simulink model "NetworkModelSimpleIntersectionCRCA"  (R2018b)
settings: Solver=VariableStepAuto  StartTime=tStart  StopTime=tFinal  FixedStep=0.001  RelTol=1e-3
values from neighbouring files (symbols this model uses):
  Ax = [0 1  0   0 ... (first row only)    [DroneSubsystemModelling.m]
  Ay = [0 1  0   0 ... (first row only)    [DroneSubsystemModelling.m]
  Bx = [0;0;0;b1]    [DroneSubsystemModelling.m]
  By = [0;0;0;b2]    [DroneSubsystemModelling.m]
  ConflictDrone2andDrone4 = ControlDetectionFunction(tout,PositionXDrone2, PositionYDrone2, PositionXDrone4, PositionYDrone4, ConflictDrone2andDrone4)    [ConflictDetection.m]    (also in ConflictDetectionTEST.m = ControlDetectionFunction(tout,PositionXDrone2TEST, PositionY)
  Cpx = [1 0 0 0]    [DroneSubsystemModelling.m]
  Cpy = [1 0 0 0]    [DroneSubsystemModelling.m]
  Cvx = [0 1 0 0]    [DroneSubsystemModelling.m]
  Cvy = [0 1 0 0]    [DroneSubsystemModelling.m]
  theta2 = -3*180/4    (= -135)    [MotionModelling.m]
  theta4 = -180/4    (= -45)    [MotionModelling.m]
  VelocityStarX2 = vx20    [MotionModelling.m]
  VelocityStarX4 = vx40    [MotionModelling.m]
  VelocityStarY2 = vy20    [MotionModelling.m]
  VelocityStarY4 = vy40    [MotionModelling.m]
  X20 = [x20 vx20 0 0]'    [MotionModelling.m]
  X40 = [x40 vx40 0 0]'    [MotionModelling.m]
  Y20 = [y20 vy20 0 0]'    [MotionModelling.m]
  Y40 = [y40 vy40 0 0]'    [MotionModelling.m]
libraries: simulink x4
settings Model: Creator=CowUser  LastModifiedBy=CowUser

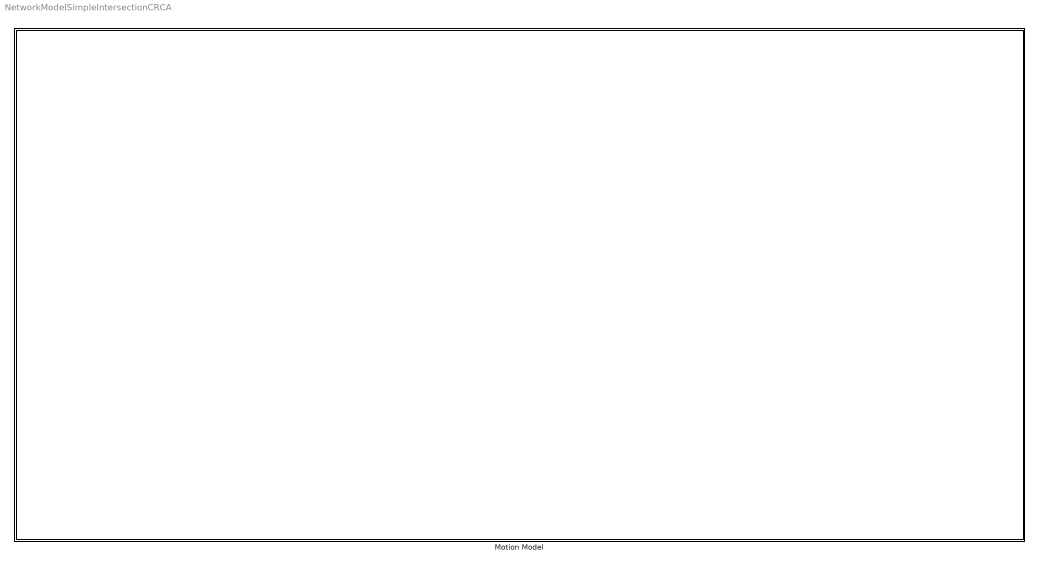
== system NetworkModelSimpleIntersectionCRCA ==
  Motion Model : Subsystem

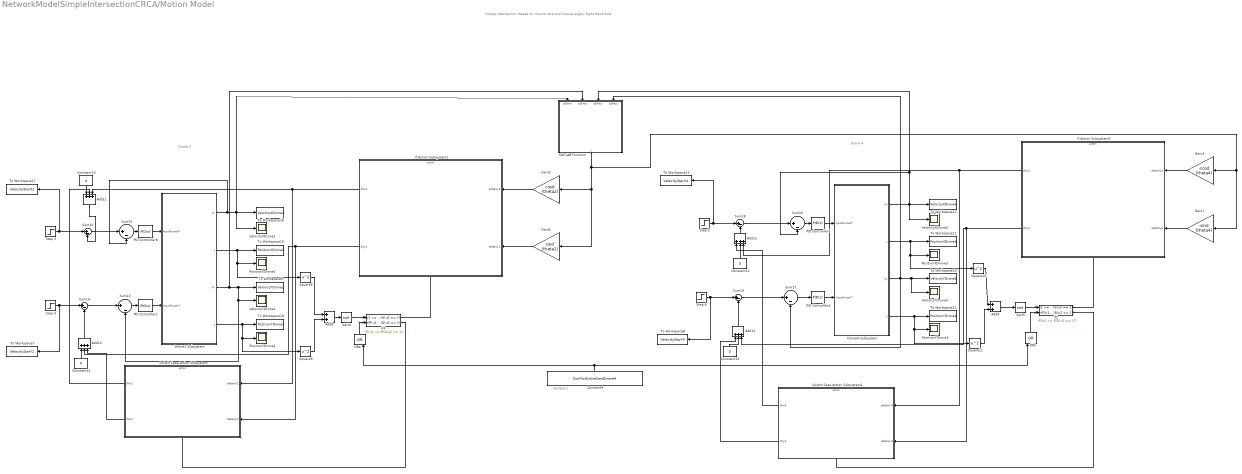
== system NetworkModelSimpleIntersectionCRCA/Motion Model ==
  note: Drone 4
  note: Drone 2
  note: Sample 1
  note: Simple Intersection
      | (based on closure rate and closure angle)
      |
      | Right Hand Rule
  Add{10..13} (4 alike) : Sum  Inputs=+++
  Add8 : Sum
  Add9 : Sum
  Constant{10..13} (4 alike) : Constant  Value=0
  Constant9 : Constant  Value=ConflictDrone2andDrone4
  Drone2 Subsystem : Subsystem
  Drone4 Subsystem : Subsystem
  Gain1 : Gain  Gain=-sind (theta4)
  Gain2 : Gain  Gain=cosd (theta2)
  Gain3 : Gain  Gain=-cosd (theta4)
  Gain4 : Gain  Gain=sind (theta2)
  If Action Subsystem2 : Subsystem  TreatAsAtomicUnit=on
  If Action Subsystem3 : Subsystem  TreatAsAtomicUnit=on
  If2 : If  NumInputs=2  IfExpression=(u1 <= R)&(u2 == 1)  ElseIfExpressions=(u1 > R)&(u2 == 1)  ShowElse=off
  If4 : If  NumInputs=2  IfExpression=(u1 <= R)&(u2 == 1)  ElseIfExpressions=(u1 > R)&(u2 == 1)  ShowElse=off
  MATLAB Function : MATLAB Function  TreatAsAtomicUnit=on
  OR3 : Logic  Operator=OR  Inputs=3  IconShape=distinctive  AllPortsSameDT=off  OutDataTypeStr='double'
  OR4 : Logic  Operator=OR  Inputs=3  IconShape=distinctive  AllPortsSameDT=off  OutDataTypeStr='double'
  PID Controller{2,4..5,8} (4 alike) : simulink/Continuous/PID Controller  Controller=PID  Form=Parallel  TimeDomain=Continuous-time  SampleTime=-1  IntegratorMethod=Forward Euler  FilterMethod=Forward Euler  ControllerParametersSource=internal  P=1.97139727738968e-05  I=1.5233344900537e-08  D=0.00566857635684116  UseFilter=on  N=15.1370363747334  TunerSelectOption=Transfer Function Based (PID Tuner App)  InitialConditionSource=internal  InitialConditionForIntegrator=0  InitialConditionForFilter=0  DifferentiatorICPrevScaledInput=0  ExternalReset=none  TrackingMode=off  Kt=1  LimitOutput=off  UpperSaturationLimit=inf  LowerSaturationLimit=-inf  LinearizeAsGain=on  AntiWindupMode=none  Kb=1  POutMin=[]  POutMax=[]  IOutMin=[]  IOutMax=[]  DOutMin=[]  DOutMax=[]  NOutMin=[]  NOutMax=[]  SumOutMin=[]  SumOutMax=[]  SaturationOutMin=[]  SaturationOutMax=[]  PParamMin=[]  PParamMax=[]  IParamMin=[]  IParamMax=[]  DParamMin=[]  DParamMax=[]  NParamMin=[]  NParamMax=[]  KbParamMin=[]  KbParamMax=[]  KtParamMin=[]  KtParamMax=[]  KbOutMin=[]  KbOutMax=[]  KtOutMin=[]  KtOutMax=[]  IntegratorOutMin=[]  IntegratorOutMax=[]  FilterOutMin=[]  FilterOutMax=[]  SumI1OutMin=[]  SumI1OutMax=[]  SumI2OutMin=[]  SumI2OutMax=[]  SumI3OutMin=[]  SumI3OutMax=[]  SumI4OutMin=[]  SumI4OutMax=[]  SumDOutMin=[]  SumDOutMax=[]  DifferentiatorOutMin=[]  DifferentiatorOutMax=[]  FilterDiffOutCoefMin=[]  FilterDiffOutCoefMax=[]  ReciprocalOutMin=[]  ReciprocalOutMax=[]  SumDenOutMin=[]  SumDenOutMax=[]  SumNumOutMin=[]  SumNumOutMax=[]  DivideOutMin=[]  DivideOutMax=[]  IntegratorContinuousStateAttributes=''  IntegratorStateMustResolveToSignalObject=off  IntegratorRTWStateStorageClass=Auto  FilterContinuousStateAttributes=''  FilterStateMustResolveToSignalObject=off  FilterRTWStateStorageClass=Auto  ParallelPVariant=InternalParameters  IdealPVariant=Disabled  IVariant=InternalParameters  DVariant=InternalParameters  IntegratorVariant=Continuous  SatVariant=Disabled  AWVariant=Passthrough  PCopyVariant=Disabled  TRVariant=Disabled  FdbkBlocksVariant=Forward  IdealPFdbkVariant=Disabled  SatFdbkVariant=Disabled  DerivativeFilterVariant=ContFilter  NVariant=InternalParameters  NCopyVariant=Disabled  FilterICVariant=InternalICsFilter  IntegratorICVariant=InternalICs  ExternalResetVariant=Disabled  TRSumVariant=Passthrough  SumFdbkVariant=Disabled  SumVariant=Sum_PID
  PositionXDrone1 : Scope
  PositionXDrone3 : Scope
  PositionYDrone1 : Scope
  PositionYDrone3 : Scope
  Sqrt4 : Sqrt  SaturateOnIntegerOverflow=on
  Sqrt5 : Sqrt  SaturateOnIntegerOverflow=on
  Square{8..11} (4 alike) : Math  Operator=square  SaturateOnIntegerOverflow=on
  Step 3 : Step  Time=0  After=VelocityStarX2  SampleTime=0
  Step 4 : Step  Time=0  After=VelocityStarY2  SampleTime=0
  Step 5 : Step  Time=0  After=VelocityStarX4  SampleTime=0
  Step 6 : Step  Time=0  After=VelocityStarY4  SampleTime=0
  Sum{13..20} (8 alike) : Sum  Inputs=|+-
  Switch Case Action Subsystem : Subsystem  TreatAsAtomicUnit=on
  Switch Case Action Subsystem1 : Subsystem  TreatAsAtomicUnit=on
  To Workspace10 : ToWorkspace  VariableName=VelocityYDrone4  SampleTime=-1
  To Workspace11 : ToWorkspace  VariableName=PositionXDrone4  SampleTime=-1
  To Workspace12 : ToWorkspace  VariableName=VelocityXDrone4  SampleTime=-1
  To Workspace13 : ToWorkspace  VariableName=VelocityStarX4  SampleTime=-1
  To Workspace14 : ToWorkspace  VariableName=PositionYDrone4  SampleTime=-1
  To Workspace15 : ToWorkspace  VariableName=PositionXDrone2  SampleTime=-1
  To Workspace16 : ToWorkspace  VariableName=VelocityXDrone2  SampleTime=-1
  To Workspace17 : ToWorkspace  VariableName=VelocityStarX2  SampleTime=-1
  To Workspace18 : ToWorkspace  VariableName=PositionYDrone2  SampleTime=-1
  To Workspace7 : ToWorkspace  VariableName=VelocityStarY2  SampleTime=-1
  To Workspace8 : ToWorkspace  VariableName=VelocityStarY4  SampleTime=-1
  To Workspace9 : ToWorkspace  VariableName=VelocityYDrone2  SampleTime=-1
  VelocityXDrone1 : Scope
  VelocityXDrone3 : Scope
  VelocityYDrone1 : Scope
  VelocityYDrone3 : Scope
  wires:
  Square10/1 -> Add9/1
  PID Controller2/1 -> Drone2 Subsystem/2("InputForceY* ")
  Sqrt4/1 -> If4/1
  Step 6/1 -> To Workspace8/1, Sum19/1
  Sum15/1 -> PID Controller8/1
  Gain2/1 -> If Action Subsystem2/1(deltaVx2)
  Step 4/1 -> Sum14/1, To Workspace7/1
  Constant9/1 -> OR4/3, OR3/1
  If Action Subsystem2/2(dVy2) -> Add10/2, Switch Case Action Subsystem/2(deltaVy2)
  Sqrt5/1 -> If2/1
  Sum16/1 -> PID Controller5/1
  If Action Subsystem3/1(dVx4) -> Switch Case Action Subsystem1/1(deltaVx4), Add12/3
  Constant10/1 -> Add11/2
  Constant13/1 -> Add13/2
  If Action Subsystem3/2(dVy4) -> Switch Case Action Subsystem1/2(deltaVy4), Add13/3
  Sum20/1 -> Sum15/1
  Add10/1 -> Sum14/2
  Drone2 Subsystem/3(Vy) -> To Workspace9/1, Sum13/2, VelocityYDrone1/1, MATLAB Function/2(qDotxj)
  PID Controller5/1 -> Drone4 Subsystem/1(InputForceX*)
  Switch Case Action Subsystem/2(dVy2) -> Add10/3
  Switch Case Action Subsystem/1(dVx2) -> Add11/1
  If4/1 -> If Action Subsystem2/Action
  Step 3/1 -> Sum20/1, To Workspace17/1
  Add11/1 -> Sum20/2
  Sum19/1 -> Sum17/1
  Sum14/1 -> Sum13/1
  Gain3/1 -> If Action Subsystem3/1(deltaVx4)
  Constant11/1 -> Add10/1
  Gain4/1 -> If Action Subsystem2/2(deltaVy2)
  OR4/1 -> If4/2
  Step 5/1 -> Sum18/1, To Workspace13/1
  Constant12/1 -> Add12/2
  Drone4 Subsystem/4(y) -> Square11/1, PositionYDrone3/1, To Workspace14/1
  If2/2 -> Switch Case Action Subsystem1/Action
  Square9/1 -> Add8/2
  Square8/1 -> Add8/1
  Add9/1 -> Sqrt5/1
  Switch Case Action Subsystem1/2(dVy4) -> Add13/1
  Sum17/1 -> PID Controller4/1
  Square11/1 -> Add9/2
  If2/1 -> If Action Subsystem3/Action
  Add13/1 -> Sum19/2
  Sum13/1 -> PID Controller2/1
  PID Controller8/1 -> Drone2 Subsystem/1(InputForceX*)
  OR3/1 -> If2/2
  If4/2 -> Switch Case Action Subsystem/Action
  Add12/1 -> Sum18/2
  Drone4 Subsystem/2(x) -> Square10/1, PositionXDrone3/1, To Workspace11/1
  Gain1/1 -> If Action Subsystem3/2(deltaVy4)
  Add8/1 -> Sqrt4/1
  Drone2 Subsystem/2(x) -> Square8/1, PositionXDrone1/1, To Workspace15/1
  MATLAB Function/1(y) -> Gain4/1, Gain2/1, Gain3/1, Gain1/1
  Drone4 Subsystem/1(Vx) -> MATLAB Function/3(qDotyi), Sum16/2, To Workspace12/1, VelocityXDrone3/1
  If Action Subsystem2/1(dVx2) -> Switch Case Action Subsystem/1(deltaVx2), Add11/3
  Drone2 Subsystem/4(y) -> To Workspace18/1, Square9/1, PositionYDrone1/1
  PID Controller4/1 -> Drone4 Subsystem/2("InputForceY* ")
  Drone4 Subsystem/3(Vy) -> MATLAB Function/4(qDotyj), Sum17/2, VelocityYDrone3/1, To Workspace10/1
  Sum18/1 -> Sum16/1
  Switch Case Action Subsystem1/1(dVx4) -> Add12/1
  Drone2 Subsystem/1(Vx) -> Sum15/2, MATLAB Function/1(qDotxi), VelocityXDrone1/1, To Workspace16/1

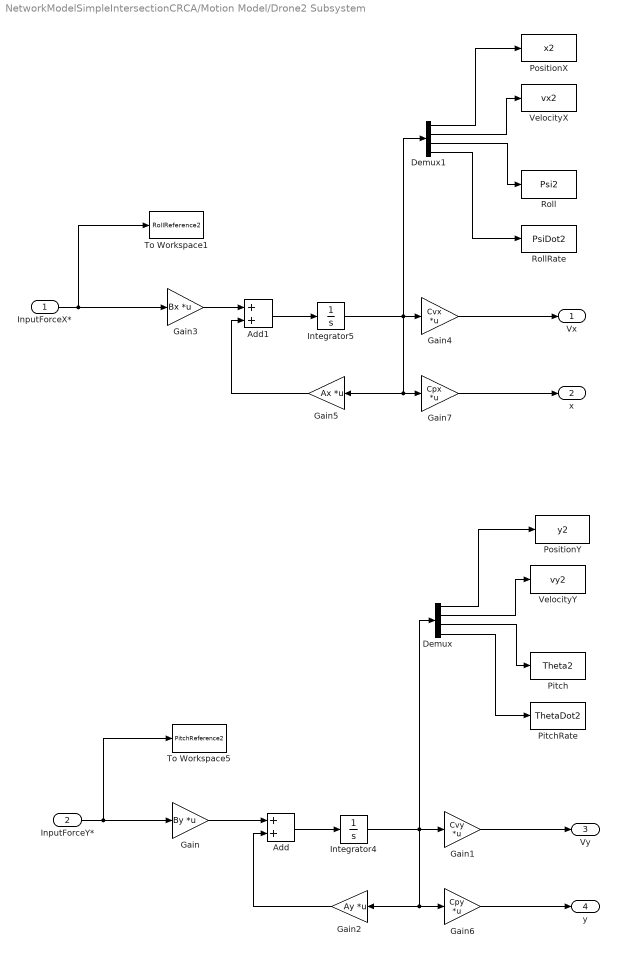
== system NetworkModelSimpleIntersectionCRCA/Motion Model/Drone2 Subsystem ==
  InputForceX* : Inport
  "InputForceY* " : Inport  Port=2
  Add : Sum
  Add1 : Sum
  Demux : Demux
  Demux1 : Demux
  Gain : Gain  Gain=By  Multiplication=Matrix(K*u)
  Gain1 : Gain  Gain=Cvy  Multiplication=Matrix(K*u)
  Gain2 : Gain  Gain=Ay  Multiplication=Matrix(K*u)
  Gain3 : Gain  Gain=Bx  Multiplication=Matrix(K*u)
  Gain4 : Gain  Gain=Cvx  Multiplication=Matrix(K*u)
  Gain5 : Gain  Gain=Ax  Multiplication=Matrix(K*u)
  Gain6 : Gain  Gain=Cpy  Multiplication=Matrix(K*u)
  Gain7 : Gain  Gain=Cpx  Multiplication=Matrix(K*u)
  Integrator4 : Integrator  InitialCondition=Y20
  Integrator5 : Integrator  InitialCondition=X20
  Pitch : ToWorkspace  VariableName=Theta2  SampleTime=-1
  PitchRate : ToWorkspace  VariableName=ThetaDot2  SampleTime=-1
  PositionX : ToWorkspace  VariableName=x2  SampleTime=-1
  PositionY : ToWorkspace  VariableName=y2  SampleTime=-1
  Roll : ToWorkspace  VariableName=Psi2  SampleTime=-1
  RollRate : ToWorkspace  VariableName=PsiDot2  SampleTime=-1
  To Workspace1 : ToWorkspace  VariableName=RollReference2  SampleTime=-1
  To Workspace5 : ToWorkspace  VariableName=PitchReference2  SampleTime=-1
  VelocityX : ToWorkspace  VariableName=vx2  SampleTime=-1
  VelocityY : ToWorkspace  VariableName=vy2  SampleTime=-1
  Vx : Outport
  x : Outport  Port=2
  Vy : Outport  Port=3
  y : Outport  Port=4
  wires:
  Demux/1 -> PositionY/1
  Demux1/2 -> VelocityX/1
  Demux1/4 -> RollRate/1
  Demux1/3 -> Roll/1
  Gain4/1 -> Vx/1
  "InputForceY* "/1 -> Gain/1, To Workspace5/1
  Gain/1 -> Add/1
  Demux/4 -> PitchRate/1
  Demux/3 -> Pitch/1
  Add/1 -> Integrator4/1
  Demux1/1 -> PositionX/1
  Gain1/1 -> Vy/1
  InputForceX*/1 -> Gain3/1, To Workspace1/1
  Gain7/1 -> x/1
  Integrator4/1 -> Gain6/1, Gain2/1, Demux/1, Gain1/1
  Demux/2 -> VelocityY/1
  Gain6/1 -> y/1
  Gain3/1 -> Add1/1
  Add1/1 -> Integrator5/1
  Gain2/1 -> Add/2
  Integrator5/1 -> Gain4/1, Gain5/1, Gain7/1, Demux1/1
  Gain5/1 -> Add1/2

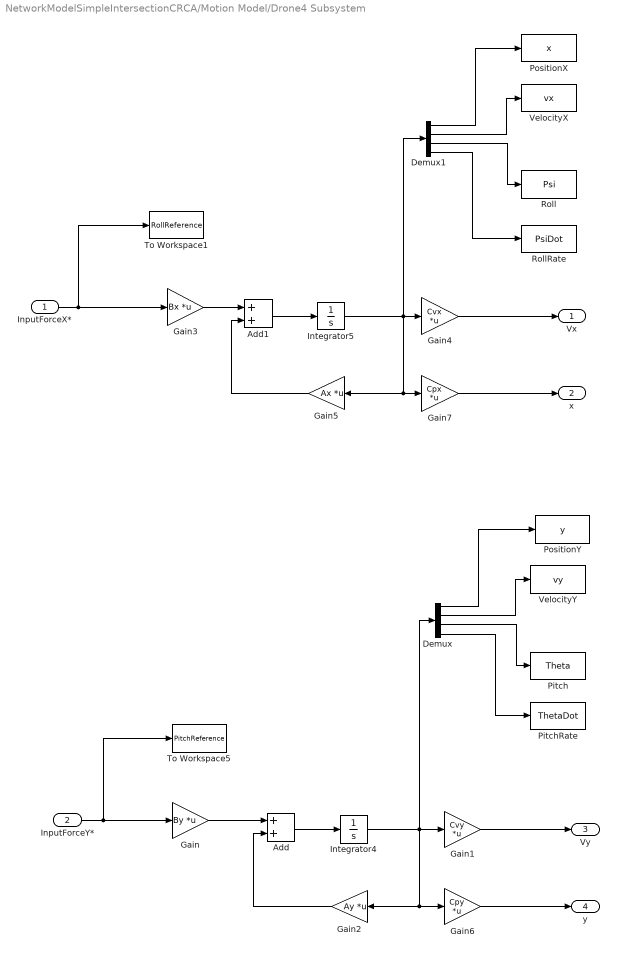
== system NetworkModelSimpleIntersectionCRCA/Motion Model/Drone4 Subsystem ==
  InputForceX* : Inport
  "InputForceY* " : Inport  Port=2
  Add : Sum
  Add1 : Sum
  Demux : Demux
  Demux1 : Demux
  Gain : Gain  Gain=By  Multiplication=Matrix(K*u)
  Gain1 : Gain  Gain=Cvy  Multiplication=Matrix(K*u)
  Gain2 : Gain  Gain=Ay  Multiplication=Matrix(K*u)
  Gain3 : Gain  Gain=Bx  Multiplication=Matrix(K*u)
  Gain4 : Gain  Gain=Cvx  Multiplication=Matrix(K*u)
  Gain5 : Gain  Gain=Ax  Multiplication=Matrix(K*u)
  Gain6 : Gain  Gain=Cpy  Multiplication=Matrix(K*u)
  Gain7 : Gain  Gain=Cpx  Multiplication=Matrix(K*u)
  Integrator4 : Integrator  InitialCondition=Y40
  Integrator5 : Integrator  InitialCondition=X40
  Pitch : ToWorkspace  VariableName=Theta  SampleTime=-1
  PitchRate : ToWorkspace  VariableName=ThetaDot  SampleTime=-1
  PositionX : ToWorkspace  VariableName=x  SampleTime=-1
  PositionY : ToWorkspace  VariableName=y  SampleTime=-1
  Roll : ToWorkspace  VariableName=Psi  SampleTime=-1
  RollRate : ToWorkspace  VariableName=PsiDot  SampleTime=-1
  To Workspace1 : ToWorkspace  VariableName=RollReference  SampleTime=-1
  To Workspace5 : ToWorkspace  VariableName=PitchReference  SampleTime=-1
  VelocityX : ToWorkspace  VariableName=vx  SampleTime=-1
  VelocityY : ToWorkspace  VariableName=vy  SampleTime=-1
  Vx : Outport
  x : Outport  Port=2
  Vy : Outport  Port=3
  y : Outport  Port=4
  wires:
  Gain4/1 -> Vx/1
  Demux/2 -> VelocityY/1
  Demux/4 -> PitchRate/1
  Gain3/1 -> Add1/1
  InputForceX*/1 -> Gain3/1, To Workspace1/1
  Gain2/1 -> Add/2
  Demux1/3 -> Roll/1
  Gain7/1 -> x/1
  Add1/1 -> Integrator5/1
  Demux/3 -> Pitch/1
  Gain5/1 -> Add1/2
  Gain6/1 -> y/1
  Integrator5/1 -> Gain4/1, Gain5/1, Gain7/1, Demux1/1
  Gain/1 -> Add/1
  Demux/1 -> PositionY/1
  Add/1 -> Integrator4/1
  Demux1/4 -> RollRate/1
  "InputForceY* "/1 -> Gain/1, To Workspace5/1
  Integrator4/1 -> Gain6/1, Gain2/1, Demux/1, Gain1/1
  Demux1/1 -> PositionX/1
  Demux1/2 -> VelocityX/1
  Gain1/1 -> Vy/1

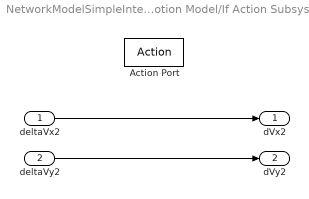
== system NetworkModelSimpleIntersectionCRCA/Motion Model/If Action Subsystem2 ==
  deltaVx2 : Inport
  deltaVy2 : Inport  Port=2
  Action Port : ActionPort  ActionType=then
  dVx2 : Outport
  dVy2 : Outport  Port=2
  wires:
  deltaVx2/1 -> dVx2/1
  deltaVy2/1 -> dVy2/1

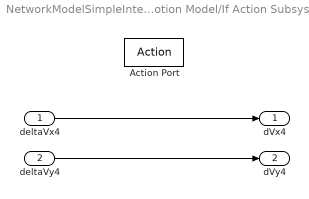
== system NetworkModelSimpleIntersectionCRCA/Motion Model/If Action Subsystem3 ==
  deltaVx4 : Inport
  deltaVy4 : Inport  Port=2
  Action Port : ActionPort  ActionType=then
  dVx4 : Outport
  dVy4 : Outport  Port=2
  wires:
  deltaVx4/1 -> dVx4/1
  deltaVy4/1 -> dVy4/1

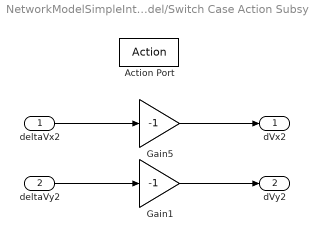
== system NetworkModelSimpleIntersectionCRCA/Motion Model/Switch Case Action Subsystem ==
  deltaVx2 : Inport
  deltaVy2 : Inport  Port=2
  Action Port : ActionPort  ActionType=elseif
  Gain1 : Gain  Gain=-1
  Gain5 : Gain  Gain=-1
  dVx2 : Outport
  dVy2 : Outport  Port=2
  wires:
  deltaVy2/1 -> Gain1/1
  deltaVx2/1 -> Gain5/1
  Gain5/1 -> dVx2/1
  Gain1/1 -> dVy2/1

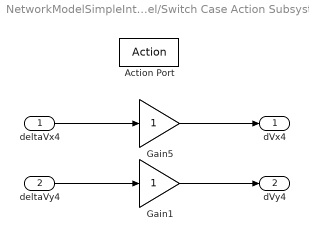
== system NetworkModelSimpleIntersectionCRCA/Motion Model/Switch Case Action Subsystem1 ==
  deltaVx4 : Inport
  deltaVy4 : Inport  Port=2
  Action Port : ActionPort  ActionType=elseif
  Gain1 : Gain
  Gain5 : Gain
  dVx4 : Outport
  dVy4 : Outport  Port=2
  wires:
  deltaVy4/1 -> Gain1/1
  deltaVx4/1 -> Gain5/1
  Gain5/1 -> dVx4/1
  Gain1/1 -> dVy4/1

== matlab function NetworkModelSimpleIntersectionCRCA/Motion Model/MATLAB Function ==
  data: qDotxi input; y output; qDotxj input; qDotyi input; qDotyj input
function y = ClosureRate(qDotxi, qDotxj, qDotyi, qDotyj)

Vmax = 0.2;
K = 1;
Vdiff = K*sqrt((qDotxi - qDotxj)^2 + (qDotyi - qDotyj)^2); 

if abs(Vdiff)>=Vmax/2
    Vdiff = Vmax/2;
end 

y = Vdiff;
